simulink model "rtwdemo_tflmuldiv"  (Simulink 7.6)
settings: Solver=FixedStepDiscrete  StartTime=0.0  StopTime=20  FixedStep=.01  RelTol=1e-3  SampleTimeConstraint=Specified
PreLoadFcn:
  | addpath(fullfile(matlabroot,'toolbox','rtw','rtwdemos','tfl_demo'));
  | sl_refresh_customizations;
libraries: rtwdemowidgets x2
settings Model: Creator=The MathWorks Inc.  ExtModeAutoUpdateStatusClock=off
settings MATStruct: SampleTime=1  Offset=0  Priority=[30.0]
settings DataIOCC: SaveOutput=off  SaveTime=off  SignalLoggingName=sigsOut
settings OptimizationCC: InlineParams=on  InlineInvariantSignals=on  PassReuseOutputArgsAs=Individual arguments  StateBitsets=on  DataBitsets=on  UseTempVars=on  ZeroExternalMemoryAtStartup=off  ZeroInternalMemoryAtStartup=off  NoFixptDivByZeroProtection=on  EfficientFloat2IntCast=on  EfficientMapNaN2IntZero=off  OptimizeModelRefInitCode=on  LifeSpan=1
settings DebuggingCC: CheckExecutionContextPreStartOutputMsg=on  CheckExecutionContextRuntimeOutputMsg=on  SolverPrmCheckMsg=none  IntegerOverflowMsg=none  StrictBusMsg=ErrorOnBusTreatedAsVector
settings HardwareCC: ProdIntDivRoundTo=Zero  ProdEndianess=LittleEndian  ProdHWDeviceType=Generic->32-bit Embedded Processor  TargetHWDeviceType=32-bit Generic
settings SFSimCC: SFSimEnableDebug=off  SFSimOverflowDetection=off  SimParseCustomCode=off
settings RTWCC: SystemTargetFile=ert.tlc  GenCodeOnly=on  TemplateMakefile=ert_default_tmf  Description=Real-Time Workshop Embedded Coder (no auto configuration)  GenerateReport=on  RTWVerbose=off  ProcessScript=ert_make_rtw_hook  IncludeHyperlinkInReport=on  LaunchReport=on
settings CodeAppCC: ForceParamTrailComments=on  IgnoreCustomStorageClasses=off  IgnoreTestpoints=on  SimulinkDataObjDesc=on  CustomSymbolStrGlobalVar=rt$N$M  CustomSymbolStrType=$N$M  CustomSymbolStrFcn=$N$M$F  CustomSymbolStrMacro=$N$M  InsertBlockDesc=on
settings ERTTargetCC: TargetFunctionLibrary=Multiplication & Division Examples  MultiwordLength=2048  GenerateSampleERTMain=on  IncludeMdlTerminateFcn=off  SupportAbsoluteTime=off  SupportNonFinite=off  SupportComplex=off  PurelyIntegerCode=on  InlinedParameterPlacement=NonHierarchical  ERTCustomFileTemplate=example_file_process.tlc  ConvertIfToSwitch=off

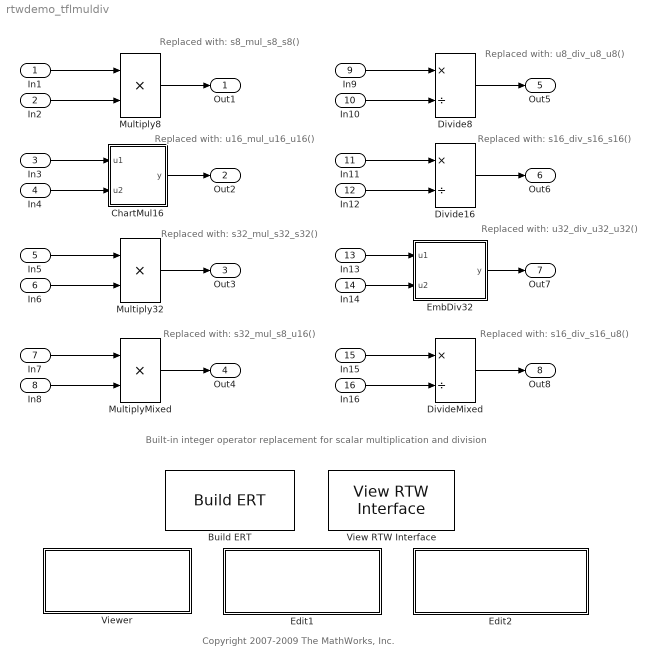
== system rtwdemo_tflmuldiv ==
  note: Copyright 2007-2009 The MathWorks, Inc.
  note: Replaced with:
      | s8_mul_s8_s8()
  note: Replaced with:
      | u16_mul_u16_u16()
  note: Replaced with:
      | s32_mul_s32_s32()
  note: Replaced with:
      | s32_mul_s8_u16()
  note: Replaced with:
      | u8_div_u8_u8()
  note: Replaced with:
      | s16_div_s16_s16()
  note: Replaced with:
      | u32_div_u32_u32()
  note: Replaced with:
      | s16_div_s16_u8()
  note: Built-in integer operator replacement for scalar multiplication and division
  In1 : Inport  OutDataTypeStr=int8  PortDimensions=1  SampleTime=1
  In2 : Inport  Port=2  OutDataTypeStr=int8  PortDimensions=1  SampleTime=1
  In3 : Inport  Port=3  OutDataTypeStr=uint16  PortDimensions=1  SampleTime=1
  In4 : Inport  Port=4  OutDataTypeStr=uint16  PortDimensions=1  SampleTime=1
  In5 : Inport  Port=5  OutDataTypeStr=int32  PortDimensions=1  SampleTime=1
  In6 : Inport  Port=6  OutDataTypeStr=int32  PortDimensions=1  SampleTime=1
  In7 : Inport  Port=7  OutDataTypeStr=int8  PortDimensions=1  SampleTime=1
  In8 : Inport  Port=8  OutDataTypeStr=uint16  PortDimensions=1  SampleTime=1
  In9 : Inport  Port=9  OutDataTypeStr=uint8  PortDimensions=1  SampleTime=1
  In10 : Inport  Port=10  OutDataTypeStr=uint8  PortDimensions=1  SampleTime=1
  In11 : Inport  Port=11  OutDataTypeStr=int16  PortDimensions=1  SampleTime=1
  In12 : Inport  Port=12  OutDataTypeStr=int16  PortDimensions=1  SampleTime=1
  In13 : Inport  Port=13  OutDataTypeStr=uint32  PortDimensions=1  SampleTime=1
  In14 : Inport  Port=14  OutDataTypeStr=uint32  PortDimensions=1  SampleTime=1
  In15 : Inport  Port=15  OutDataTypeStr=int16  PortDimensions=1  SampleTime=1
  In16 : Inport  Port=16  OutDataTypeStr=uint8  PortDimensions=1  SampleTime=1
  Build ERT : rtwdemowidgets/Build ERT  SystemSampleTime=-1  attrib_overrides={'GenFloatMathFcnCalls'}
  ChartMul16 : Stateflow chart  TreatAsAtomicUnit=on
  Divide16 : Product  Inputs=*/  OutDataTypeStr=int16  RndMeth=Nearest
  Divide8 : Product  Inputs=*/  OutDataTypeStr=uint8
  DivideMixed : Product  Inputs=*/  OutDataTypeStr=int16  RndMeth=Zero
  Edit1 : Subsystem  mask{attrib_overrides={}}
      mask prompts: attrib_overrides "List of attributes to preserve (cell of strings):"
      mask help: Enter the attributes of the configuration set that you want preserved. Otherwise, the default configuration script will override your current settings.
      settings: OpenFcn=edit('tfl_table_muldiv');
      mask Display:
      | disp(['View/edit TFL Definition\n',...
      | 	  'tfl_table_muldiv.m\n(double-click)'])
  Edit2 : Subsystem  mask{attrib_overrides={}}
      mask prompts: attrib_overrides "List of attributes to preserve (cell of strings):"
      mask help: Enter the attributes of the configuration set that you want preserved. Otherwise, the default configuration script will override your current settings.
      settings: OpenFcn=edit(fullfile(matlabroot,'toolbox','rtw','rtwdemos','tfl_demo', 'sl_customization.m'));
      mask Display:
      | disp(['View/edit TFL Registration\n',...
      | 	  'sl_customization.m\n(double-click)'])
  EmbDiv32 : Stateflow chart  TreatAsAtomicUnit=on
  Multiply32 : Product  OutDataTypeStr=int32  SaturateOnIntegerOverflow=on  RndMeth=Zero
  Multiply8 : Product  OutDataTypeStr=int8  SaturateOnIntegerOverflow=on  RndMeth=Zero
  MultiplyMixed : Product  OutDataTypeStr=int32  RndMeth=Zero
  View RTW Interface : rtwdemowidgets/View RTW Interface  SystemSampleTime=-1
  Viewer : Subsystem  mask{attrib_overrides={}}
      mask prompts: attrib_overrides "List of attributes to preserve (cell of strings):"
      mask help: Enter the attributes of the configuration set that you want preserved. Otherwise, the default configuration script will override your current settings.
      settings: OpenFcn=|
      | tfl = tfl_table_muldiv;
      | obj = RTW.viewTfl(tfl);
      | clear tfl obj;
      mask Display:
      | disp(['Invoke TFL Viewer on\n',...
      | 	  'tfl_table_muldiv.m\n(double-click)'])
  Out1 : Outport
  Out2 : Outport  Port=2
  Out3 : Outport  Port=3
  Out4 : Outport  Port=4
  Out5 : Outport  Port=5
  Out6 : Outport  Port=6
  Out7 : Outport  Port=7
  Out8 : Outport  Port=8
  wires:
  Multiply8/1 -> Out1/1
  In1/1 -> Multiply8/1
  In2/1 -> Multiply8/2
  ChartMul16/1(y) -> Out2/1
  In3/1 -> ChartMul16/1(u1)
  In4/1 -> ChartMul16/2(u2)
  Multiply32/1 -> Out3/1
  In5/1 -> Multiply32/1
  In6/1 -> Multiply32/2
  MultiplyMixed/1 -> Out4/1
  In7/1 -> MultiplyMixed/1
  In8/1 -> MultiplyMixed/2
  Divide8/1 -> Out5/1
  In9/1 -> Divide8/1
  In10/1 -> Divide8/2
  Divide16/1 -> Out6/1
  In11/1 -> Divide16/1
  In12/1 -> Divide16/2
  EmbDiv32/1(y) -> Out7/1
  In13/1 -> EmbDiv32/1(u1)
  In14/1 -> EmbDiv32/2(u2)
  DivideMixed/1 -> Out8/1
  In15/1 -> DivideMixed/1
  In16/1 -> DivideMixed/2

== system rtwdemo_tflmuldiv/Edit1 ==

== system rtwdemo_tflmuldiv/Edit2 ==

== system rtwdemo_tflmuldiv/Viewer ==

== stateflow chart ChartMul16 ==
  (default) -> (junction 3) : {y := u1*u2;}
  data: u1 input uint16; u2 input uint16; y output uint16

== matlab function EmbDiv32 ==
  data: u1 input uint32; y output uint32; u2 input uint32
function y = fcn(u1, u2)
% This block supports the Embedded MATLAB subset.
% See the help menu for details. 

assert(isa(u1,'uint32'));
assert(isa(u2,'uint32'));

if (u2 ~= 0)
    y = idivide(u1,u2);
else
    y = intmax('uint32');
end
